simulink model "Q8_simulation"  (R2017b)
settings: Solver=VariableStepAuto  StartTime=0.0  StopTime=8  RelTol=1e-3
settings Model: Creator=ACER  LastModifiedBy=HeMaTshop

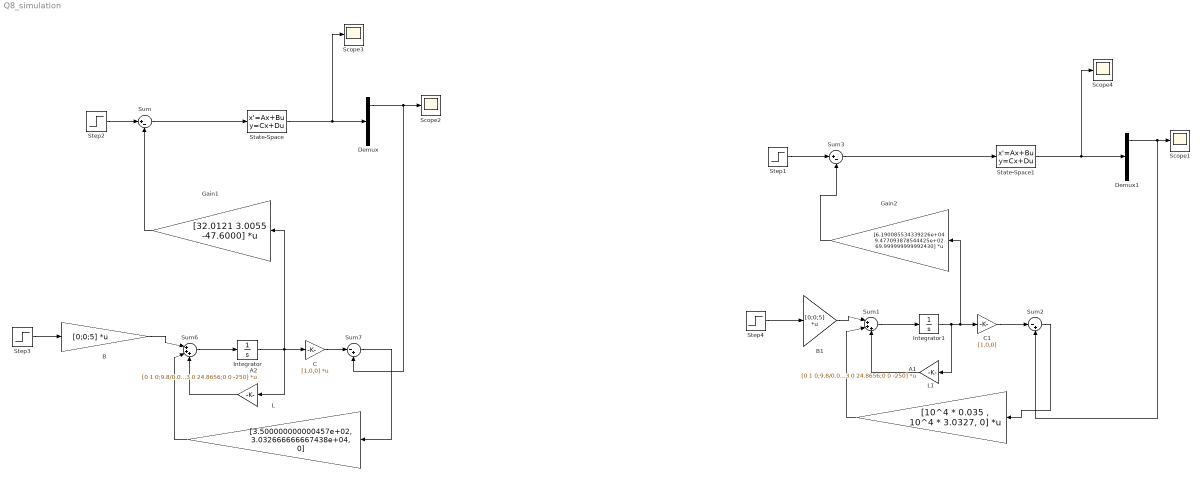
== system Q8_simulation ==
  A1 : Gain  Gain=[0 1 0;9.8/0.03 0 24.8656;0 0 -250]  Multiplication=Matrix(K*u)
  A2 : Gain  Gain=[0 1 0;9.8/0.03 0 24.8656;0 0 -250]  Multiplication=Matrix(K*u)
  B : Gain  Gain=[0;0;5]  Multiplication=Matrix(K*u)
  B1 : Gain  Gain=[0;0;5]  Multiplication=Matrix(K*u)
  C : Gain  Gain=[1,0,0]  Multiplication=Matrix(K*u)
  C1 : Gain  Gain=[1,0,0]
  Demux : Demux  Outputs=3
  Demux1 : Demux  Outputs=3
  Gain1 : Gain  Gain="[32.0121    3.0055  -47.6000]"  Multiplication=Matrix(K*u)
  Gain2 : Gain  Gain="[6.190085534339226e+04    9.477093878544425e+02  69.999999999992430]"  Multiplication=Matrix(K*u)
  Integrator : Integrator
  Integrator1 : Integrator
  L : Gain  Gain=[3.500000000000457e+02, 3.032666666667438e+04, 0]
  L1 : Gain  Gain=[10^4 * 0.035 , 10^4 * 3.0327, 0]  Multiplication=Matrix(K*u)
  Scope{1..4} (4 alike) : Scope
  State-Space : StateSpace  A=[0 1 0;9.8/0.03 0 24.8656;0 0 -250]  B=[0;0;5]  C=eye(3)  D=[0;0;0]  InitialCondition=0
  State-Space1 : StateSpace  A=[0 1 0;9.8/0.03 0 24.8656;0 0 -250]  B=[0;0;5]  C=eye(3)  D=[0;0;0]  InitialCondition=0
  Step{1..4} (4 alike) : Step  Time=0  SampleTime=0
  Sum : Sum  Inputs=|+-
  Sum1 : Sum  Inputs=|+++
  Sum2 : Sum  Inputs=|-+
  Sum3 : Sum  Inputs=|+-
  Sum6 : Sum  Inputs=|+++
  Sum7 : Sum  Inputs=|-+
  wires:
  Demux/1 -> Scope2/1, Sum7/2
  State-Space/1 -> Scope3/1, Demux/1
  Sum6/1 -> Integrator/1
  Integrator/1 -> Gain1/1, A2/1, C/1
  C/1 -> Sum7/1
  Sum7/1 -> L/1
  L/1 -> Sum6/2
  Step3/1 -> B/1
  B/1 -> Sum6/1
  C1/1 -> Sum2/1
  B1/1 -> Sum1/1
  Integrator1/1 -> A1/1, Gain2/1, C1/1
  Sum2/1 -> L1/1
  A1/1 -> Sum1/3
  Demux1/1 -> Sum2/2, Scope1/1
  Step4/1 -> B1/1
  L1/1 -> Sum1/2
  Sum1/1 -> Integrator1/1
  State-Space1/1 -> Scope4/1, Demux1/1
  A2/1 -> Sum6/3
  Gain1/1 -> Sum/2
  Step2/1 -> Sum/1
  Sum/1 -> State-Space/1
  Gain2/1 -> Sum3/2
  Step1/1 -> Sum3/1
  Sum3/1 -> State-Space1/1
